simulink model "F4PhantomRemodel"  (R2023b)
settings: Solver=VariableStepAuto  StartTime=0.0  StopTime=10.0  RelTol=1e-3
values from neighbouring files (symbols this model uses):
  alpha1 = 2.6    [F4ModelCode.m]    (also in F4ModelCodeV2.m; F4ModelCodeV2Q2PartD.m; F4PhantomModelCode.m)
  c_D_delta_E = 0    [F4ModelCode.m]    (also in F4ModelCodeV2.m; F4ModelCodeV2Q2PartD.m; F4PhantomModelCode.m)
  c_D_i = -0.10    (= -0.1)    [F4PhantomModelCode.m]
  cbar_ft = 16.0    (= 16)    [F4ModelCode.m]    (also in F4ModelCodeV2.m; F4ModelCodeV2Q2PartD.m; F4PhantomModelCode.m)
  FTx = 0    [F4ModelCode.m]    (also in F4ModelCodeV2.m; F4ModelCodeV2Q2PartD.m)
  fTx = 0    [F4ModelCode.m]    (also in F4ModelCodeV2.m; F4ModelCodeV2Q2PartD.m)
  FTy = 0    [F4ModelCode.m]    (also in F4ModelCodeV2.m; F4ModelCodeV2Q2PartD.m)
  fTy = 0    [F4ModelCode.m]    (also in F4ModelCodeV2.m; F4ModelCodeV2Q2PartD.m)
  FTz = 0    [F4ModelCode.m]    (also in F4ModelCodeV2.m; F4ModelCodeV2Q2PartD.m)
  fTz = 0    [F4ModelCode.m]    (also in F4ModelCodeV2.m; F4ModelCodeV2Q2PartD.m)
  g = -32.2    [F4ModelCode.m]    (also in F4ModelCodeV2.m; F4ModelCodeV2Q2PartD.m; F4PhantomModelCode.m)
  i_H = zeros(length(timeVec),1)    [F4ModelCode.m]    (also in F4ModelCodeV2.m; F4ModelCodeV2Q2PartD.m; F4PhantomModelCode.m = 0)
  LT = 0    [F4ModelCode.m]    (also in F4ModelCodeV2Q2PartD.m)
  lT = 0    [F4ModelCode.m]    (also in F4ModelCodeV2Q2PartD.m)
  Mach = 0.9    [F4ModelCode.m]    (also in F4ModelCodeV2.m; F4ModelCodeV2Q2PartD.m; F4PhantomModelCode.m)
  mass = Weight/32.2    (= 1211.18012422)    [F4ModelCode.m]    (also in F4ModelCodeV2.m; F4ModelCodeV2Q2PartD.m; F4PhantomModelCode.m = 1212.157)
  MT = 0    [F4ModelCode.m]    (also in F4ModelCodeV2Q2PartD.m)
  mT = 0    [F4ModelCode.m]    (also in F4ModelCodeV2Q2PartD.m)
  NT = 0    [F4ModelCode.m]    (also in F4ModelCodeV2Q2PartD.m)
  nT = 0    [F4ModelCode.m]    (also in F4ModelCodeV2Q2PartD.m)
  q0 = angle2quat(phidot,thetadot,psidot)    [F4ModelCode.m]    (also in F4ModelCodeV2.m; F4ModelCodeV2Q2PartD.m)
  qbar1 = 283.2    [F4ModelCode.m]    (also in F4ModelCodeV2.m; F4ModelCodeV2Q2PartD.m; F4PhantomModelCode.m)
  S_ft2 = 530    [F4ModelCode.m]    (also in F4ModelCodeV2.m; F4ModelCodeV2Q2PartD.m; F4PhantomModelCode.m)
  uv = Mach*a    (= 871.2)    [F4ModelCode.m]    (also in F4ModelCodeV2.m; F4ModelCodeV2Q2PartD.m; F4PhantomModelCode.m)
  Weight = 39000    [F4ModelCode.m]    (also in F4ModelCodeV2.m; F4ModelCodeV2Q2PartD.m; F4PhantomModelCode.m)
undefined symbols (not defined in the file or in its folder): t_max
libraries: shared6dof x1
settings Model: Creator=Owner  LastModifiedBy=Owner

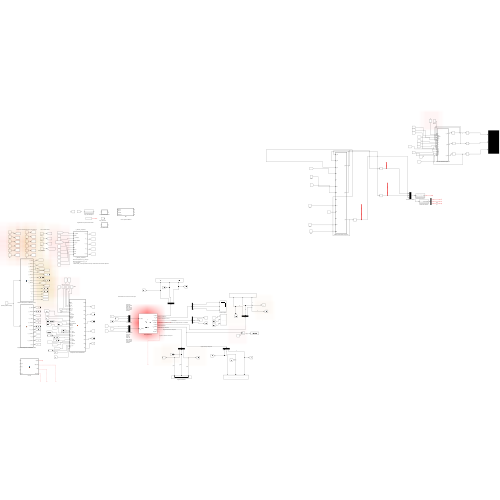
[thumbnail: Simulink's stored preview of the top-level diagram]
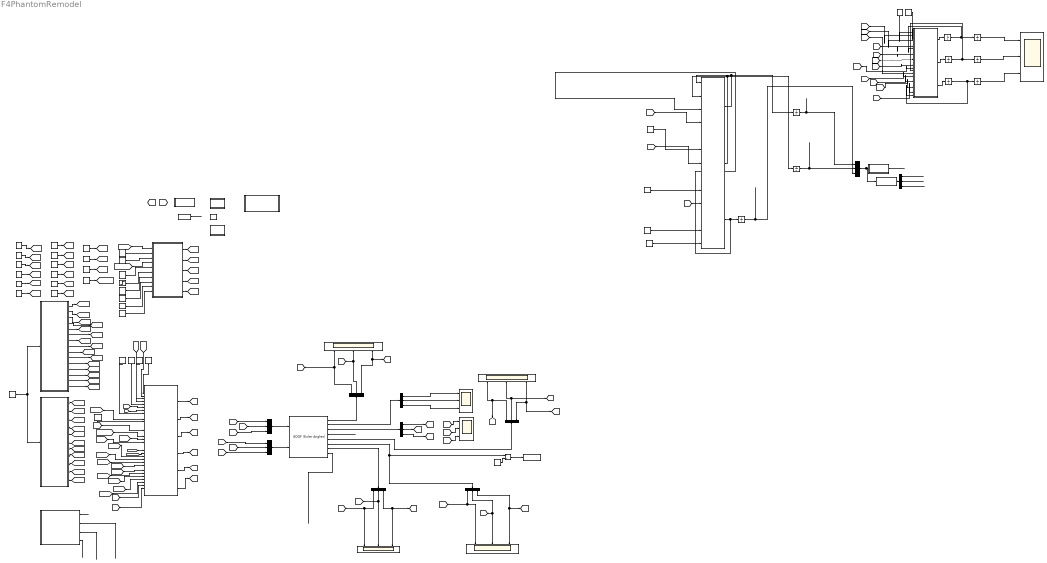
== system F4PhantomRemodel ==
  note: Don't have equation for c_D_delta_E?
      | Don't have equation for c_D_i_H?
      | - c_D_i was given
      | - need to make i_H an array based of time step. variable names are within the step block
  note: c_Attribute_1 Equations
  note: Thrust Force and Moment Inputs (=0 for project 1)
  note: Control Surface Inputs
  note: Future Equations Needed
  note: These Need to be moved to the correct spot
  note: Copy Blocks to be placed where needed
  note: Create the moment functions within this block, fed be a vector or array of the needed variables
  note: Create the force functions within this block, fed be a vector or array of the needed variables
  6DOF (Quaternion) : shared6dof/6DOF (Euler Angles)  units=English (Velocity in ft/s)  mtype=Fixed  rep=Quaternion  xme_0=InitialInertialPosition  Vm_0=InitialVelocity  eul_0=InitialEulerOrientation  pm_0=InitialRotationRates  mass_0=1.0  mass_e=0.5  mass_f=2.0  inertia=eye(3)  inertia_e=eye(3)  inertia_f=2*eye(3)  k_quat=1.0  vre_flag=on  abi_flag=off  aMode=0  xme_statename=''  Vm_statename=''  eul_statename=''  quat_statename=''  pm_statename=''  mass_statename=''
      settings: LibrarySourceBlock=aerolib6dof2/6DOF (Quaternion)
  Aerodynamic Forces and Moments : MATLAB Function  TreatAsAtomicUnit=on
  Aerodynamic Paramaters : MATLAB Function  TreatAsAtomicUnit=on
  Aircraft Trajectory : Scope  NumInputPorts=3
  Angular Acceleration : Scope  NumInputPorts=3
  CAME Perturbed Motion Equations : MATLAB Function  TreatAsAtomicUnit=on
  CLME Perturbed Motion Equations : MATLAB Function  TreatAsAtomicUnit=on
  Constant : Constant  Value=alpha1
  Constant1 : Constant  Value=alpha1
  Constant11 : Constant  Value=uv
  Constant12 : Constant  Value=alpha1
  Constant2 : Constant  Value=c_D_delta_E
  Constant3 : Constant  Value=c_D_i
  Constant4 : Constant  Value=Weight
  Constant5 : Constant  Value=qbar1
  Constant6 : Constant  Value=S_ft2
  Constant7 : Constant  Value=Mach
  Copy This Function : MATLAB Function  TreatAsAtomicUnit=on
  Copy This SubSystem : Subsystem
  Copy This block : Constant
  Demux{,1..6} (7 alike) : Demux  Outputs=3
  Divide : Product  Inputs=*/  Multiplication=Matrix(*)
  Euler Kinematic Eqs : Subsystem
  FTx : Constant  Value=FTx
  FTy : Constant  Value=FTy
  FTz : Constant  Value=FTz
  Force Vector : Mux  Inputs=3
  From File : FromFile  SampleTime=0
  From6 : From
  Goto9 : Goto
  IKE : MATLAB Function  TreatAsAtomicUnit=on
  "IXX " : Constant
  IXZ : Constant
  IYY : Constant
  IZZ : Constant
  InputArray (Need to Assign) : Constant
  Integrator{1..3,12..17} (9 alike) : Integrator
  LT : Constant  Value=LT
  "Latitudinal Aerodynamic Coeffiecents (HW4) " : MATLAB Function  TreatAsAtomicUnit=on
  Longitudinal Aerodynamic Coeffiecents (HW3) : MATLAB Function  TreatAsAtomicUnit=on
  MT : Constant  Value=MT
  Mass : Constant  Value=mass
  Moment Vector : Mux  Inputs=3
  NT : Constant  Value=NT
  Quaternion Rotations : Subsystem
  S_ft2 : Constant  Value=S_ft2
  Scope{,1..4} (5 alike) : Scope  NumInputPorts=3
  Step : Step  Time=t  Before=i_H  After=t_max  SampleTime=0
  To Quaternion Matrix : Mux  Inputs=3
  To Workspace : ToWorkspace  VariableName=simout  SaveFormat=Timeseries  SampleTime=-1
  c_Attribute_1 Equations : MATLAB Function  TreatAsAtomicUnit=on
  cbar_ft : Constant  Value=cbar_ft
  delta_A : Constant
  delta_E : Constant
  delta_R : Constant
  delta_Stabilitator : Constant
  fTx : Constant  Value=fTx
  fTy : Constant  Value=fTy
  fTz : Constant  Value=fTz
  g : Constant  Value=g
  lT : Constant  Value=lT
  mT : Constant  Value=mT
  nT : Constant  Value=nT
  qbar1 : Constant  Value=qbar1
  α and β : MATLAB Function  TreatAsAtomicUnit=on
  wires:
  Force Vector/1 -> 6DOF (Quaternion)/1
  From File/1 -> ?
  CLME Perturbed Motion Equations/1(u_dot) -> Integrator12/1
  CLME Perturbed Motion Equations/3(w_dot) -> Integrator14/1
  CLME Perturbed Motion Equations/2(v_dot) -> Integrator13/1
  Integrator12/1 -> CLME Perturbed Motion Equations/8(u), Integrator15/1  "u"
  Integrator13/1 -> CLME Perturbed Motion Equations/16(v), Integrator16/1  "v"
  Integrator14/1 -> CLME Perturbed Motion Equations/25(w), Integrator17/1  "w"
  Integrator16/1 -> Scope1/2  "y"
  Integrator15/1 -> Scope1/1  "x"
  Integrator17/1 -> Scope1/3  "z"
  6DOF (Quaternion)/1 -> Demux3/1  "Velocity in Inertial Axes"
  6DOF (Quaternion)/2 -> Demux2/1  "Position in Inertial Axes (X' Y' Z')"
  6DOF (Quaternion)/3 -> Demux1/1  "Euler Angles"
  6DOF (Quaternion)/4 -> ?  "Coordinate Transformation from Flat Earth axes to Body-Fixed axes in a 3x3 Matrix"
  6DOF (Quaternion)/5 -> Demux6/1  "Velocity in Body Axes"
  6DOF (Quaternion)/6 -> Demux5/1, Divide/1  "Angular Velocity for Body Axes"
  6DOF (Quaternion)/7 -> Demux4/1  "Angular Acceleration for Body Axes"
  6DOF (Quaternion)/8 -> ?  "Angular Acceleration for Body Axes"
  InputArray (Need to Assign)/1 -> Longitudinal Aerodynamic Coeffiecents (HW3)/1(u), "Latitudinal Aerodynamic Coeffiecents (HW4) "/1(u)
  Aerodynamic Forces and Moments/2(fAx) -> [fAx]
  [fAx] -> CLME Perturbed Motion Equations/18(fAx)
  Aerodynamic Forces and Moments/4(fAz) -> [fAz]
  [fAz] -> CLME Perturbed Motion Equations/22(fAz)
  Aerodynamic Forces and Moments/6(fAy) -> [fAy]
  [fAy] -> CLME Perturbed Motion Equations/20(fAy)
  Mass/1 -> CLME Perturbed Motion Equations/1(m)
  g/1 -> CLME Perturbed Motion Equations/2(g)
  Longitudinal Aerodynamic Coeffiecents (HW3)/1(c_L_alpha) -> [c_L_alpha]
  [c_L_alpha] -> Aerodynamic Forces and Moments/22(c_L_alpha)
  Longitudinal Aerodynamic Coeffiecents (HW3)/2(c_L_delta_E) -> [c_L_delta_E]
  [c_L_delta_E] -> Aerodynamic Forces and Moments/25(c_L_delta_E)
  Longitudinal Aerodynamic Coeffiecents (HW3)/3(c_L_i_H) -> [c_L_i_H]
  [c_L_i_H] -> Aerodynamic Forces and Moments/26(c_L_i_H)
  Longitudinal Aerodynamic Coeffiecents (HW3)/4(c_m_alpha) -> [c_m_alpha]
  [c_m_alpha] -> Aerodynamic Forces and Moments/28(c_m_alpha)
  Longitudinal Aerodynamic Coeffiecents (HW3)/5(c_m_delta_E) -> [c_m_delta_E]
  [c_m_delta_E] -> Aerodynamic Forces and Moments/31(c_m_delta_E)
  [c_m_i_H] -> Aerodynamic Forces and Moments/32(c_m_i_H)
  Longitudinal Aerodynamic Coeffiecents (HW3)/7(c_m_i_H) -> [c_m_i_H]
  Longitudinal Aerodynamic Coeffiecents (HW3)/8(c_L_alphadot) -> [c_L_alphadot]
  [c_L_alphadot] -> Aerodynamic Forces and Moments/23(c_L_alphadot)
  Longitudinal Aerodynamic Coeffiecents (HW3)/9(c_L_q) -> [c_L_q]
  [c_L_q] -> Aerodynamic Forces and Moments/24(c_L_q)
  Longitudinal Aerodynamic Coeffiecents (HW3)/10(c_m_alphadot) -> [c_m_alphadot]
  [c_m_alphadot] -> Aerodynamic Forces and Moments/29(c_m_alphadot)
  Longitudinal Aerodynamic Coeffiecents (HW3)/11(c_m_q) -> [c_m_q]
  [c_m_q] -> Aerodynamic Forces and Moments/30(c_m_q)
  qbar1/1 -> Aerodynamic Forces and Moments/1(qbar1)
  S_ft2/1 -> Aerodynamic Forces and Moments/3(S_ft2)
  cbar_ft/1 -> Aerodynamic Forces and Moments/5(cbar_ft)
  Constant11/1 -> Aerodynamic Forces and Moments/8(uv)
  Constant12/1 -> Aerodynamic Forces and Moments/11(alpha_deg)
  Moment Vector/1 -> 6DOF (Quaternion)/2
  [fAz] -> Force Vector/2
  [fAx] -> Force Vector/1
  Aerodynamic Forces and Moments/10(mA) -> [mA]
  [mA] -> Moment Vector/2
  Aerodynamic Forces and Moments/12(nA) -> [nA]
  Aerodynamic Forces and Moments/8(lA) -> [lA]
  [fAy] -> Force Vector/3
  [nA] -> Moment Vector/3
  [lA] -> Moment Vector/1
  CAME Perturbed Motion Equations/1(p_dot) -> CAME Perturbed Motion Equations/1("p_dot "), Integrator1/1
  CAME Perturbed Motion Equations/2(q_dot) -> CAME Perturbed Motion Equations/2("q_dot "), Integrator2/1
  CAME Perturbed Motion Equations/3(r_dot) -> CAME Perturbed Motion Equations/3("r_dot "), Integrator3/1
  Integrator3/1 -> To Quaternion Matrix/3  "r"
  Integrator2/1 -> To Quaternion Matrix/2  "q"
  Integrator1/1 -> To Quaternion Matrix/1  "p"
  "Latitudinal Aerodynamic Coeffiecents (HW4) "/1(c_Y_beta) -> [c_Y_beta]
  "Latitudinal Aerodynamic Coeffiecents (HW4) "/2(c_Y_delta_A) -> [c_Y_delta_A]
  "Latitudinal Aerodynamic Coeffiecents (HW4) "/3(c_Y_delta_R) -> [c_Y_delta_R]
  "Latitudinal Aerodynamic Coeffiecents (HW4) "/4(c_n_beta) -> [c_n_beta]
  "Latitudinal Aerodynamic Coeffiecents (HW4) "/5(c_n_delta_A) -> [c_n_delta_A]
  "Latitudinal Aerodynamic Coeffiecents (HW4) "/6(c_n_delta_R) -> [c_n_delta_R]
  "Latitudinal Aerodynamic Coeffiecents (HW4) "/7(c_l_beta) -> [c_l_beta]
  "Latitudinal Aerodynamic Coeffiecents (HW4) "/8(c_l_delta_A) -> [c_l_delta_A]
  "Latitudinal Aerodynamic Coeffiecents (HW4) "/9(c_l_delta_R) -> [c_l_delta_R]
  "Latitudinal Aerodynamic Coeffiecents (HW4) "/10(c_l_p) -> [c_l_p]
  "Latitudinal Aerodynamic Coeffiecents (HW4) "/11(c_Y_p) -> [c_Y_p]
  "Latitudinal Aerodynamic Coeffiecents (HW4) "/12(c_n_p) -> [c_n_p]
  "Latitudinal Aerodynamic Coeffiecents (HW4) "/13(c_l_r) -> [c_l_r]
  "Latitudinal Aerodynamic Coeffiecents (HW4) "/15(c_n_r) -> [c_n_r]
  "Latitudinal Aerodynamic Coeffiecents (HW4) "/14(c_Y_r) -> [c_Y_r]
  [p] -> CLME Perturbed Motion Equations/10(p)
  IZZ/1 -> CAME Perturbed Motion Equations/13(IZZ)
  IXZ/1 -> CAME Perturbed Motion Equations/12(IXZ)
  IYY/1 -> CAME Perturbed Motion Equations/9(IYY)
  "IXX "/1 -> CAME Perturbed Motion Equations/6(IXX)
  [lA] -> CAME Perturbed Motion Equations/4(lA)
  [nA] -> CAME Perturbed Motion Equations/10(nA)
  [mA] -> CAME Perturbed Motion Equations/7(mA)
  [q] -> CLME Perturbed Motion Equations/12(q)
  [r] -> CLME Perturbed Motion Equations/14(r)
  To Quaternion Matrix/1 -> Quaternion Rotations/1(In1), Euler Kinematic Eqs/1(In1)
  Euler Kinematic Eqs/1(Phi) -> ?
  Quaternion Rotations/1(Euler Angles) -> Demux/1
  Demux/3 -> ?  "psi"
  Demux/2 -> ?  "theta"
  Demux/1 -> ?
  Demux1/1 -> [phi]  "phi"
  Demux1/2 -> [theta]  "theta"
  Demux1/3 -> [psi]  "psi"
  [phi] -> Scope/1
  [theta] -> Scope/2
  [psi] -> Scope/3
  Demux2/1 -> Aircraft Trajectory/1  "X'"
  Demux2/2 -> Aircraft Trajectory/2  "Y'"
  Demux2/3 -> Aircraft Trajectory/3  "Z'"
  Demux3/1 -> Scope3/1, [U1]
  Demux3/2 -> [V1], Scope3/2
  Demux3/3 -> Scope3/3, [W1]
  [U1] -> CLME Perturbed Motion Equations/7(U1)
  [V1] -> CLME Perturbed Motion Equations/15(V1)
  [W1] -> CLME Perturbed Motion Equations/24(W1)
  Demux4/1 -> [r_dot], Angular Acceleration/1  "r_dot"
  Demux4/2 -> [q_dot], Angular Acceleration/2  "q_dot"
  Demux4/3 -> [p_dot], Angular Acceleration/3  "p_dot"
  Demux5/1 -> [r], Scope4/1  "r"
  Demux5/2 -> [q], Scope4/2  "q"
  Demux5/3 -> [p], Scope4/3  "p"
  Constant/1 -> Divide/2
  Divide/1 -> To Workspace/1  "V_P_1"
  delta_Stabilitator/1 -> [delta_Stabilitator]
  delta_A/1 -> [delta_A]
  delta_R/1 -> [delta_R]
  delta_E/1 -> [delta_E]
  [delta_Stabilitator] -> Aerodynamic Forces and Moments/16(delta_Stabilitator)
  [delta_A] -> Aerodynamic Forces and Moments/17(delta_A)
  [delta_R] -> Aerodynamic Forces and Moments/18(delta_R)
  [q] -> Aerodynamic Forces and Moments/14(q)
  Longitudinal Aerodynamic Coeffiecents (HW3)/6(c_D_alpha) -> [c_D_alpha]
  [c_D_alpha] -> Aerodynamic Forces and Moments/10(c_D_alpha)
  [theta] -> CLME Perturbed Motion Equations/3(theta)
  [phi] -> CLME Perturbed Motion Equations/5(phi)
  [psi] -> CLME Perturbed Motion Equations/17(psi)
  fTz/1 -> [fTz]
  fTy/1 -> [fTy]
  fTx/1 -> [fTx]
  FTz/1 -> [FTz]
  FTy/1 -> [FTy]
  FTx/1 -> [FTx]
  LT/1 -> [LT]
  MT/1 -> [MT]
  NT/1 -> [NT]
  lT/1 -> [lT]
  mT/1 -> [mT]
  nT/1 -> [nT]
  [p] -> Aerodynamic Forces and Moments/33(p)
  [r] -> Aerodynamic Forces and Moments/34(r)
  Constant1/1 -> c_Attribute_1 Equations/2(alpha1)
  [c_D_alpha] -> c_Attribute_1 Equations/1(c_D_alpha)
  Constant2/1 -> c_Attribute_1 Equations/3(c_D_delta_E)
  [delta_Stabilitator] -> c_Attribute_1 Equations/4(delta_stabilitator)
  Step/1 -> c_Attribute_1 Equations/6(i_H)
  Constant3/1 -> c_Attribute_1 Equations/5(c_D_i_H)
  Constant4/1 -> c_Attribute_1 Equations/7(W)
  Constant5/1 -> c_Attribute_1 Equations/8(qbar1)
  Constant6/1 -> c_Attribute_1 Equations/9(S_ft2)
  Constant7/1 -> c_Attribute_1 Equations/10(Mach)
  c_Attribute_1 Equations/1(c_D_1) -> [c_D_1]
  c_Attribute_1 Equations/2(c_L_1) -> [c_L_1]
  c_Attribute_1 Equations/3(c_m_1) -> [c_m_1]
  c_Attribute_1 Equations/4(c_L_u) -> [c_L_u]
  c_Attribute_1 Equations/5(c_D_u) -> [c_D_u]
  [c_D_1] -> Aerodynamic Forces and Moments/2(c_D_1)
  [c_L_1] -> Aerodynamic Forces and Moments/4(c_L_1)
  [c_m_1] -> Aerodynamic Forces and Moments/6(c_m_1)
  [c_D_u] -> Aerodynamic Forces and Moments/7(c_D_u)
  α and β/1(alpha1) -> ?
  α and β/4(beta_dot) -> ?
  α and β/3(beta) -> ?
  α and β/2(alpha_dot) -> ?
  [c_L_u] -> Aerodynamic Forces and Moments/21(c_L_u)
  Demux6/3 -> [V], Scope2/3  "V"
  Demux6/2 -> [W], Scope2/2  "W"
  Demux6/1 -> Scope2/1, [U]  "U"

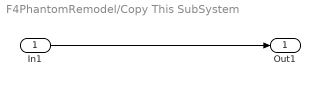
== system F4PhantomRemodel/Copy This SubSystem ==
  In1 : Inport
  Out1 : Outport
  wires:
  In1/1 -> Out1/1

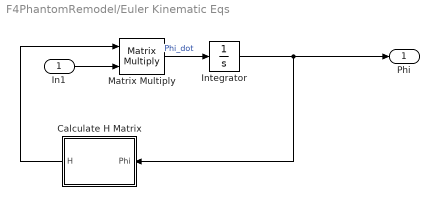
== system F4PhantomRemodel/Euler Kinematic Eqs ==
  In1 : Inport
  Calculate H Matrix : MATLAB Function  TreatAsAtomicUnit=on
  Integrator : Integrator
  Matrix Multiply : Product  Multiplication=Matrix(*)
  Phi : Outport
  wires:
  In1/1 -> Matrix Multiply/2
  Matrix Multiply/1 -> Integrator/1  "Phi_dot"
  Integrator/1 -> Calculate H Matrix/1(Phi), Phi/1
  Calculate H Matrix/1(H) -> Matrix Multiply/1

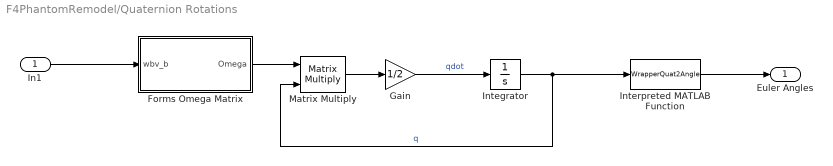
== system F4PhantomRemodel/Quaternion Rotations ==
  In1 : Inport
  Forms Omega Matrix : MATLAB Function  TreatAsAtomicUnit=on
  Gain : Gain  Gain=1/2
  Integrator : Integrator  InitialCondition=q0
  Interpreted MATLAB Function : MATLABFcn  MATLABFcn=WrapperQuat2Angle
  Matrix Multiply : Product  Multiplication=Matrix(*)
  Euler Angles : Outport
  wires:
  Interpreted MATLAB Function/1 -> Euler Angles/1
  Matrix Multiply/1 -> Gain/1
  Forms Omega Matrix/1(Omega) -> Matrix Multiply/1
  Integrator/1 -> Interpreted MATLAB Function/1, Matrix Multiply/2  "q"
  Gain/1 -> Integrator/1  "qdot"
  In1/1 -> Forms Omega Matrix/1(wbv_b)

== matlab function F4PhantomRemodel/Latitudinal Aerodynamic Coeffiecents (HW4)  ==
  data: u input; c_Y_beta output; c_Y_delta_A output; c_Y_delta_R output; c_n_beta output; c_n_delta_A output; c_n_delta_R output; c_l_beta output; c_l_delta_A output; c_l_delta_R output; c_l_p output; c_Y_p output; c_n_p output; c_l_r output; c_Y_r output; c_n_r output
function [c_Y_beta, c_Y_delta_A, c_Y_delta_R, c_n_beta, c_n_delta_A, c_n_delta_R, c_l_beta, c_l_delta_A, c_l_delta_R, c_l_p, c_Y_p, c_n_p, c_l_r, c_Y_r, c_n_r] = fcn(u)

C_Y_delta_A = 0;

C_Y_delta_R = abs(C_L_alpha_V) *eta_V*((0.5*S2V)/S_ft2)*delta_K_R*tau_R ;

C_Y_beta_W = -.0001 * ((GammaW_deg)) * 57.3 ;
C_Y_beta_H = -.0001 * abs((GammaH_deg)) * 57.3 * (.724 + 3.06 * ((S_H/S_ft2)/(1+cos(rad2deg(LambdaLE_quarter_rad))))+(.4*(ZW_ft/d_ft))+(.009*ARH)) *(S_H/S_ft2);  
C_Y_beta_B = -2*(.96*(SP_V_ft2/S_ft2));
C_Y_beta_V = -K_Y_V * abs(C_L_alpha_V_eff) * (.724 + 3.06 * ((S_V/S_ft2)/(1+cos((LambdaLE_quarter_rad))))+(.4*(ZW_ft/d_ft))+(.009*AR_V_eff)) *(S_V/S_ft2);
C_Y_beta = C_Y_beta_W + C_Y_beta_B + C_Y_beta_H  + C_Y_beta_V ;


y = u;

== matlab function F4PhantomRemodel/Longitudinal Aerodynamic Coeffiecents (HW3) ==
  data: u input; c_L_alpha output; c_L_delta_E output; c_L_i_H output; c_m_alpha output; c_m_delta_E output; c_D_alpha output; c_m_i_H output; c_L_alphadot output; c_L_q output; c_m_alphadot output; c_m_q output
function [c_L_alpha, c_L_delta_E, c_L_i_H, c_m_alpha, c_m_delta_E, c_D_alpha, c_m_i_H, c_L_alphadot, c_L_q, c_m_alphadot, c_m_q] = fcn(u)

c_L_alpha_W = c_L_alpha_W_mach;
c_L_alpha_H = c_L_alpha_H_mach*eta_H*(S_H/S_ft2)*(1-d_epsilon_dalpha_mach);
c_L_alpha = c_L_alpha_W_mach + c_L_alpha_H;

c_L_delta_E = 0; 

c_L_i_H = c_L_alpha_H_mach*eta_H*(S_H/S_ft2);

c_m_alpha = (c_L_alpha_W_mach*(xbar_CG - xbar_AC_WB)) - c_L_alpha_H_mach*eta_H*(S_H/S_ft2)*(1-d_epsilon_dalpha_mach)*(xbar_AC_H - xbar_CG);

c_m_i_H = -c_L_alpha_H_mach*eta_H*(S_H/S_ft2) * (xbar_AC_H - xbar_CG);

c_m_delta_E = c_m_i_H * tau_E;

c_D_alpha = ((2*c_L_1)/(pi*AR*e))*c_L_alpha;

c_L_alphadot = 2*c_L_alpha_H_mach*eta_H*(S_H/S_ft2)*(xbar_AC_H - xbar_CG)*(d_epsilon_dalpha_mach);

piece1 = (AR+(2*cos(LambdaLE_quarter_rad)))/(AR*(sqrt((1-Mach^2)*cos(LambdaLE_quarter_rad)^2))+(2*cos(LambdaLE_quarter_rad)));
piece2 = ((0.5+2*abs(xbar_AC_W-xbar_CG))*c_L_alpha_W_mach0);
piece3 = 2*c_L_alpha_H*eta_H*((S_H/S_ft2)*(xbar_AC_H-xbar_CG));
c_L_q = piece1+piece2+piece3;

c_m_alphadot = -2*c_L_alpha_H_mach*eta_H*(S_H/S_ft2)*((xbar_AC_H - xbar_CG)^2)*d_epsilon_dalpha_mach;

lefttopfrac = ((AR^3) * (tan(LambdaLE_quarter_rad)^2))/(AR+(6*cos(LambdaLE_quarter_rad)));
righttopfrac = 3/(sqrt((1-Mach^2)*(cos(LambdaLE_quarter_rad)^2)));
bottomfrac = (((AR^3) * (tan(LambdaLE_quarter_rad)^2))/(AR+(6*(tan(LambdaLE_quarter_rad)^2)))) +3;

secondpiece = -K_q*c_L_alpha_W_mach0*(cos(LambdaLE_quarter_rad));
thirdpiece = ((AR*(0.5*abs(xbar_AC_W-xbar_CG)+(2*abs(xbar_AC_W-xbar_CG)^2)))/(AR+(2*cos(LambdaLEH_quarter_rad)))) + (((1/24) * ((AR^3)* tan(LambdaLE_quarter_rad)^2)/(AR+(6*cos(LambdaLE_quarter_rad))))) + 1/8;
fourthpiece = -2*c_L_alpha_H_mach*eta_H*(S_H/S_ft2)*((xbar_AC_H-xbar_CG)^2) ;
frac = (lefttopfrac+righttopfrac)/(bottomfrac);
c_m_q = (frac * secondpiece * thirdpiece) + fourthpiece;

== matlab function F4PhantomRemodel/Euler Kinematic Eqs/Calculate H Matrix ==
  data: Phi input; H output
function H = fcn(Phi)

%Unpack Phi
phi     = Phi(1);
theta   = Phi(2);
psi     = Phi(3);

%Input the H matrix
H = [1 tan(theta)*sin(phi) tan(theta)*cos(phi);
    0 cos(phi) -sin(phi);
    0 sin(phi)/cos(theta) cos(phi)/cos(theta)];

== matlab function F4PhantomRemodel/Quaternion Rotations/Forms Omega Matrix ==
  data: wbv_b input; Omega output
function Omega  = fcn(wbv_b)

wx = wbv_b(1);
wy = wbv_b(2);
wz = wbv_b(3);

Omega = [0 -wx -wy -wz;
    wx 0 wz -wy;
    wy -wz 0 wx;
    wz wy -wx 0];

== matlab function F4PhantomRemodel/c_Attribute_1 Equations ==
  data: c_D_alpha input; c_D_1 output; alpha1 input; c_D_delta_E input; delta_stabilitator input; c_D_i_H input; i_H input; W input; qbar1 input; S_ft2 input; Mach input; c_L_1 output; c_m_1 output; c_L_u output; c_D_u output
function [c_D_1, c_L_1, c_m_1, c_L_u, c_D_u] = fcn(c_D_alpha, alpha1, c_D_delta_E, delta_stabilitator, c_D_i_H, i_H, W, qbar1, S_ft2, Mach)

c_D_0 = 0;

c_D_1 = c_D_0 + (c_D_alpha*alpha1) + (c_D_delta_E * delta_stabilitator) + (c_D_i_H*i_H);

c_L_1 = W/(qbar1*S_ft2);

c_m_1 = 0;

c_L_u = ((Mach^2)/(1-Mach^2))*c_L_1;

c_D_u = 0;

== matlab function F4PhantomRemodel/CAME Perturbed Motion Equations ==
  data: p_dot input; p_dot output; q_dot input; r_dot input; lA input; lT input; IXX input; mA input; mT input; IYY input; nA input; nT input; IXZ input; IZZ input; q_dot output; r_dot output
function [p_dot, q_dot, r_dot] = fcn(p_dot, q_dot, r_dot, lA, lT, IXX, mA, mT, IYY, nA, nT, IXZ, IZZ)
%CAME - Still Needs to be fixed
%P_dot = ((la+lt)+(R_dot.*IXZ)+(P.*Q.*IXZ)-((R*Q).*(IZZ-IYY)))./(IXX);
%Q_dot = ((ma+mt)-(R_dot.*IXZ)+(P.*Q.*IXZ)-(R*Q).*(IZZ-IYY))./(IYY);
%R_dot = ((nA+nT) + (P_dot*IXZ) - (((P1*q)+(p*Q1))*(IYY-IXX)) - (((Q1*r)+(R1*q))*IXZ))/(IZZ);

p_dot = ((r_dot*IXZ) + (lA+lT))/IXX;
q_dot = (mA+mT)/IYY;
r_dot = ((nA+nT) + (p_dot*IXZ))/IZZ;

%Need to reorganzie to solve for it

== matlab function F4PhantomRemodel/Aerodynamic Forces and Moments ==
  data: qbar1 input; c_D_1 input; S_ft2 input; c_L_1 input; cbar_ft input; c_m_1 input; c_D_u input; uv input; FAx output; V_P_1 input; c_D_alpha input; alpha_deg input; alphadot input; c_D_q input; q input; c_D_delta_E input; delta_Stabilitator input; delta_A input; delta_R input; c_D_i_H input; i_H input; c_L_u input; c_L_alpha input; c_L_alphadot input; c_L_q input; c_L_delta_E input; c_L_i_H input; c_m_u input; c_m_alpha input; c_m_alphadot input; c_m_q input; c_m_delta_E input; c_m_i_H input; fAx output; FAz output; fAz output; FAy output; fAy output; LA output; lA output; MA output; mA output; NA output; nA output; p input; r input
function [FAx, fAx, FAz, fAz, FAy, fAy, LA, lA, MA, mA, NA, nA]  = fcn(qbar1, c_D_1, S_ft2, c_L_1, cbar_ft, c_m_1, c_D_u, uv, V_P_1, c_D_alpha, alpha_deg, alphadot, c_D_q, q, c_D_delta_E, delta_Stabilitator, delta_A, delta_R, c_D_i_H, i_H, c_L_u, c_L_alpha, c_L_alphadot, c_L_q, c_L_delta_E, c_L_i_H, c_m_u, c_m_alpha, c_m_alphadot, c_m_q, c_m_delta_E, c_m_i_H, p, r)

FAx = -qbar1*S_ft2*c_D_1;
fAx = (qbar1*S_ft2)*(((-(c_D_u+(2*c_D_1)))*(uv/V_P_1)) + ((c_D_alpha + c_L_1)*(alpha_deg)) - c_D_alphadot*((alphadot*cbar_ft)/(2*V_P_1)) - c_D_q*((q*cbar)/(2*V_P_1)) - (c_D_delta_E*delta_Stabilitator)-(c_D_i_H*i_H));

FAz = -qbar1*S_ft2*c_L_1;
fAz = (qbar1*S_ft2)*(((-(c_L_u+(2*c_L_1)))*(uv/V_P_1)) + ((c_L_alpha + c_D_1)*(alpha_deg)) - c_L_alphadot*((alphadot*cbar_ft)/(2*V_P_1)) - c_L_q*((q*cbar)/(2*V_P_1)) - (c_L_delta_E*delta_Stabilitator)-(c_L_i_H*i_H));

FAy = -qbar1*S_ft2*c_Y_1;
fAy = -qbar1*S_ft2 * ((c_Y_beta*beta) + c_Y_betadot * ((betadot*b_ft)/(2*V_P_1)) + c_Y_p*((p*b_ft)/(2*V_P_1)) + c_Y_r * ((r*b_ft)/(2*V_P_1)) +(c_Y_delta_A * delta_A) + (c_Y_delta_R*delta_R));

LA = -qbar1*S_ft2*b_ft*c_l_1;
lA = -qbar1*S_ft2*b_ft*((c_l_beta*beta) + c_l_betadot * ((betadot*b_ft)/(2*V_P_1)) + c_l_p*((p*b_ft)/(2*V_P_1)) + c_l_r * ((r*b_ft)/(2*V_P_1)) +(c_l_delta_A * delta_A) + (c_l_delta_R*delta_R));

MA = -qbar1*S_ft2*cbar_ft*c_m_1;
mA = (qbar1*S_ft2*cbar_ft)*(((-(c_m_u+(2*c_m_1)))*(uv/V_P_1)) + (c_m_alpha*alpha_deg) + c_m_alphadot*((alphadot*cbar_ft)/(2*V_P_1)) + c_m_q*((q*cbar_ft)/(2*V_P_1)) + (c_m_delta_E*delta_Stabilitator)+(c_L_i_H*i_H));

NA = -qbar1*S_ft2*b_ft*c_n_1;
nA = -qbar1*S_ft2*b_ft*((c_n_beta*beta) + c_n_betadot * ((betadot*b_ft)/(2*V_P_1)) + c_n_p*((p*b_ft)/(2*V_P_1)) + c_n_r * ((r*b_ft)/(2*V_P_1)) +(c_n_delta_A * delta_A) + (c_n_delta_R*delta_R));

%Need to get rid of fAy and lA and nA, leave MA and mA

== matlab function F4PhantomRemodel/IKE ==
  data: phi_dot input; p output; psi_dot input; THETA1 input; theta_dot input; q output; r output
function [p,q,r] = fcn(phi_dot, psi_dot, THETA1, theta_dot)

p = (phi_dot)-(psi_dot*sind(THETA1));
q = theta_dot;
r = psi_dot*cosd(THETA1);


y = u;

== matlab function F4PhantomRemodel/α and β ==
  data: w input; alpha1 output; alpha_dot output; beta output; w_dot input; V_P_1 input; v input; v_dot input; beta_dot output
function [alpha1, alpha_dot, beta, beta_dot] = fcn(w, w_dot, V_P_1, v, v_dot)

alpha1 = w/V_P_1;

alpha_dot = w_dot/V_P_1;

beta = v/V_P_1;

beta_dot = v_dot/V_P_1;

== matlab function F4PhantomRemodel/Aerodynamic Paramaters ==
  data: u input; y output
function y = fcn(u)

y = u;

== matlab function F4PhantomRemodel/Copy This Function ==
  data: u input; y output
function y = fcn(u)

y = u;

== matlab function F4PhantomRemodel/CLME Perturbed Motion Equations ==
  data: m input; u_dot output; g input; theta input; THETA1 input; phi input; PHI1 input; U1 input; u input; P1 input; p input; Q1 input; q input; R1 input; r input; v_dot output; w_dot output; V1 input; v input; psi input; fAx input; fTx input; fAy input; fTy input; fAz input; fTz input; W1 input; w input
function [u_dot, v_dot, w_dot] = fcn(m, g, theta, THETA1, phi, PHI1, U1, u, P1, p, Q1, q, R1, r, V1, v, psi, fAx, fTx, fAy, fTy, fAz, fTz, W1, w)

%Mass = 2300; %kg
%g = 9.81; %m/s
%theta = 0;
%Fax = 0;
%Ftx = 0;

%u_dot = (1/m) * ((-m*g*theta*cosd(THETA1)) + (fAx + fTx) - (Q1*w) - (q*W1) + (R1*v) + (r*V1));
%v_dot = (1/m) * (((-m*g*theta*sind(PHI1)*sind(THETA1))+(m*g*phi*cosd(PHI1)*cosd(THETA1))) + (fAy + fTy) - (U1*r) - (u*R1) + (P1*w) + (p*W1));
%w_dot = (1/m) * (((-m*g*theta*cosd(PHI1)*sind(THETA1))-(m*g*phi*sind(PHI1)*cosd(THETA1))) + (fAz + fTz) - (P1*v) - (V1*p) + (Q1*u) + (U1*q));

u_dot = (1/m) * ((-m*g*theta*cosd(THETA1)) + (fAx + fTx) - (q*W1));
v_dot = (1/m) * ((m*g*phi*cosd(THETA1)) + (fAy+fTy) - (U1*r) + (p*W1));
w_dot = (1/m) * ((-m*g*theta*sind(THETA1)) + (fAz + fTz) + (U1*q));
